simulink model "d"  (R2012b)
settings: Solver=ode45  StartTime=0.0  StopTime=10.0  RelTol=1e-3
settings Model: Creator=ZhouHaoyu  LastModifiedBy=ZhouHaoyu

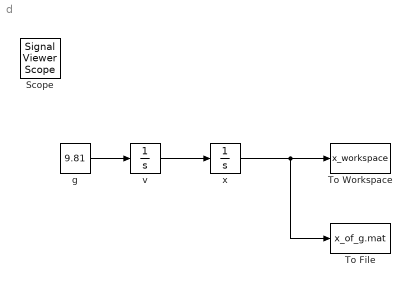
== system d ==
  To File : ToFile  Filename=x_of_g.mat  MatrixName=x_file  SaveFormat=Timeseries
  To Workspace : ToWorkspace  VariableName=x_workspace  SampleTime=-1
  g : Constant  Value=9.81
  v : Integrator
  x : Integrator
  Scope : SignalViewerScope  IOType=viewer  RefreshTime=0.035000
  wires:
  g/1 -> v/1
  v/1 -> x/1
  x/1 -> To File/1, To Workspace/1
